simulink model "robot_fis_opt_monte_carlo"  (R2023a)
settings: Solver=FixedStepDiscrete  StartTime=0.0  StopTime=200  RelTol=1e-3
model workspace (MAT data in the model file):
  x = 1
  y = [100; 100; 100; 100; 100; 100; 100; 100; 100; 100; 100; 100; 100; 100; 100; 100; 100; 100; 100; 100; 100; 95; 90; 85; 80; 75; 70; 65; 60; 55; 50; 45; 40; 35; 30; 25; 20; 15; 10; 5; 0; 0; 0; 0; 0; 0; 0; 0; 0; 0; 0; 0; 0; 0; 0; 0; 0; 0; 0; 0; 0; 0; 0; 0; 0; 0; 0; 0; 0; 0; 0; 0; 0; 0; 0; 0; 0; 0; 0; 0; 0; 0; 0; 0; 0; 0; 0; 0; 0; 0; 0; 0; 0; 0; 0; 0; 0; 0; 0; 0; 0; 0; 0; 0; 0; 0; 0; 0; 0; 0; 0; 0; 0; 0; 0; 0; 0; 0; 0; 0; 0; 0; 0; 0; 0; 0; 0; 0; 0; 0; 0; 0; 0; 0; 0; 0; 0; 0; 0; 0; 0; 0; 0; 0; 0; 0; 0; 0; 0; 0; 0; 0; 0; 0; 0; 0; 0; 0; 0; 0; 0; 0; 0; 0; 0; 0; 0; 0; 0; 0; 0; 0; 0; 0; 0; 0; 0; 0; 0; 0; 0; 0; 0; 0; 0; 0; 0; 0; 0; 0; 0; 0; 0; 0; 0; 0; 0; 0; 0; 0; 0; 0; 0; 0; 0; 0; 0; 0; 0; 0; 0; 0; 0; 0; 0; 0; 0; 0; 0; 0; 0; 0; 0; 0; 0; 0; 0; 0; 0; 0; 0; 0; 0; 0; 0; 0; 0; 0; 0; 0; 0; 0; 0; 0; 0; 0; 0; 0; 0; 0; 0; 0; 0; 0; 0; 0]
libraries: fuzblock x1
settings Model: DataTypeOverride=Off  SnapshotBufferSize=1000  SnapshotInterval=1000  Creator=Mohammad  LastModifiedBy=Mohammad
settings SolverCC: AlgebraicLoopSolver=TrustRegion
settings DataIOCC: SaveOutput=off  SaveTime=off
settings OptimizationCC: BlockReduction=off  ConditionallyExecuteInputs=off  DefaultParameterBehavior=Inlined
settings DebuggingCC: AlgebraicLoopMsg=error  SingleTaskRateTransMsg=error  UnconnectedInputMsg=warning  UnconnectedOutputMsg=warning  UnconnectedLineMsg=warning  StrictBusMsg=ErrorOnBusTreatedAsVector  ArithmeticOperatorsInVariantConditions=warning
settings HardwareCC: ProdBitPerPointer=32  ProdBitPerSizeT=32  ProdBitPerPtrDiffT=32  ProdLargestAtomicFloat=None  ProdIntDivRoundTo=Undefined  ProdEndianess=Unspecified  ProdWordSize=32  ProdHWDeviceType=ASIC/FPGA->ASIC/FPGA  ProdEqTarget=off
settings ModelReferenceCC: EnableRefExpFcnMdlSchedulingChecks=on
settings SFSimCC: SimUseLocalCustomCode=off  CustomCodeUndefinedFunction=UseInterfaceOnly
settings RTWCC: RTWUseLocalCustomCode=off
settings CodeAppCC: StateflowObjectComments=on
settings GRTTargetCC: TargetLangStandard=C89/C90 (ANSI)

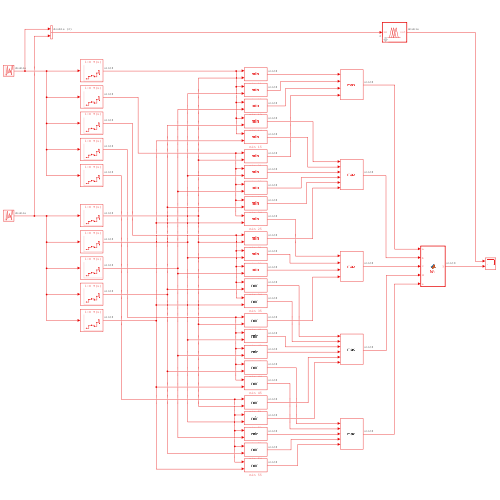
[thumbnail: Simulink's stored preview of the top-level diagram]
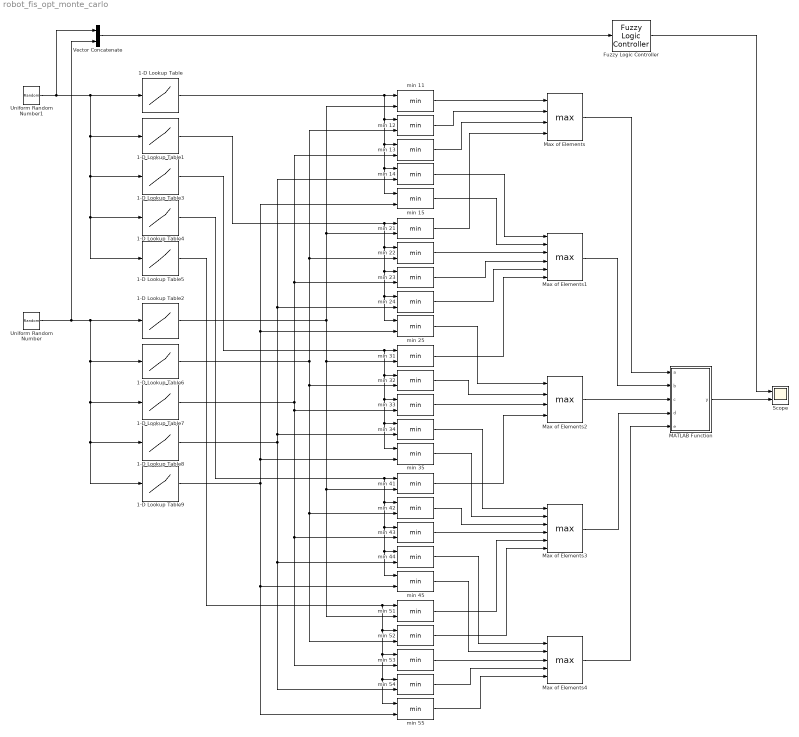
== system robot_fis_opt_monte_carlo ==
  1-D Lookup Table : Lookup_n-D  NumberOfTableDimensions=1  BreakpointsSpecification=Even spacing  BreakpointsForDimension1=[0 1 2 3 4 5 6 7]  BreakpointsForDimension1FirstPoint=0  BreakpointsForDimension1Min=0  BreakpointsForDimension1Max=255  BreakpointsForDimension1DataTypeStr=uint8  IndexSearchMethod=Linear search  Table=[100;100;100;100;100;100;100;100;100;100;100;100;100;100;100;100;100;100;100;100;100;95;90;85;80;75;70;65;64;64;50;45;40;35;30;25;20;15;10;5;0;0;0;0;0;0;0;0;0;0;0;0;0;0;0;0;0;0;0;0;0;0;0;0;0;0;0;0;0;0;0;0;0;0;0;0;0;0;0;0;0;0;0;0;0;0;0;0;0;0;0;0;0;0;0;0;0;0;0;0;0;0;0;0;0;0;0;0;0;0;0;0;0;0;0;0;0;0;0;0;0;0;0;0;0;0;0;0;0;0;0;0;0;0;0;0;0;0;0;0;0;0;0;0;0;0;0;0;0;0;0;0;0;0;0;0;0;0;0;0;0;0;0;0;0;0;0;0;0;0;0;0;0;0;0;0;0;0;0;0;0;0;0;0;0;0;0;0;0;0;0;0;0;0;0;0;0;0;0;0;0;0;0;0;0;0;0;0;0;0;0;0;0;0;0;0;0;0;0;0;0;0;0;0;0;0;0;0;0;0;0;0;0;0;0;0;0;0;0;0;0;0;0;0;0;0;0;0;0;0;0;0;0;0;0;0]  TableMin=0  TableMax=100  TableDataTypeStr=uint8  IntermediateResultsDataTypeStr=int8  InterpMethod=Flat  InternalRulePriority=Speed  OutDataTypeStr=uint8  FractionDataTypeStr=fixdt(0,8,0)
  1-D Lookup Table1 : Lookup_n-D  NumberOfTableDimensions=1  BreakpointsSpecification=Even spacing  BreakpointsForDimension1=[0 1 2 3 4 5 6 7]  BreakpointsForDimension1FirstPoint=0  BreakpointsForDimension1Min=0  BreakpointsForDimension1Max=255  BreakpointsForDimension1DataTypeStr=uint8  IndexSearchMethod=Linear search  Table=[0;0;0;0;0;0;0;0;0;0;0;0;0;0;0;0;0;0;0;0;0;5;10;15;20;25;30;35;40;45;50;55;64;65;70;75;80;85;90;95;100;100;100;100;100;100;100;100;100;100;100;100;100;100;100;100;100;100;100;100;100;95;90;85;80;75;70;65;64;64;50;45;40;35;30;25;20;15;10;5;0;0;0;0;0;0;0;0;0;0;0;0;0;0;0;0;0;0;0;0;0;0;0;0;0;0;0;0;0;0;0;0;0;0;0;0;0;0;0;0;0;0;0;0;0;0;0;0;0;0;0;0;0;0;0;0;0;0;0;0;0;0;0;0;0;0;0;0;0;0;0;0;0;0;0;0;0;0;0;0;0;0;0;0;0;0;0;0;0;0;0;0;0;0;0;0;0;0;0;0;0;0;0;0;0;0;0;0;0;0;0;0;0;0;0;0;0;0;0;0;0;0;0;0;0;0;0;0;0;0;0;0;0;0;0;0;0;0;0;0;0;0;0;0;0;0;0;0;0;0;0;0;0;0;0;0;0;0;0;0;0;0;0;0;0;0;0;0;0;0;0;0;0;0;0;0]  TableMin=0  TableMax=100  TableDataTypeStr=uint8  IntermediateResultsDataTypeStr=int8  InterpMethod=Flat  InternalRulePriority=Speed  OutDataTypeStr=uint8  FractionDataTypeStr=fixdt(0,8,0)
  1-D Lookup Table2 : Lookup_n-D  NumberOfTableDimensions=1  BreakpointsSpecification=Even spacing  BreakpointsForDimension1=[0 1 2 3 4 5 6 7]  BreakpointsForDimension1FirstPoint=0  BreakpointsForDimension1Min=0  BreakpointsForDimension1Max=1023  BreakpointsForDimension1DataTypeStr=fixdt(0,10)  IndexSearchMethod=Linear search  Table=[100;100;100;100;100;100;100;100;100;100;100;100;100;100;100;100;100;100;100;100;100;100;100;100;100;100;100;100;100;100;100;100;100;100;100;100;100;100;100;100;100;100;100;100;100;100;100;100;100;100;100;100;100;100;100;100;100;100;100;100;100;100;100;100;100;100;100;100;100;100;100;100;100;100;100;100;100;100;100;100;100;100;100;100;100;100;100;100;100;100;100;100;100;100;100;100;100;100;100;100;100;99;98;97;96;95;94;93;92;91;90;89;88;87;86;85;84;83;82;81;80;79;78;77;76;75;74;73;63;63;63;63;63;63;63;63;63;63;62;61;60;59;58;57;56;55;54;53;52;51;50;49;48;47;46;45;44;43;42;41;40;39;38;37;36;35;34;33;32;31;30;29;28;27;26;25;24;23;22;21;20;19;18;17;16;15;14;13;12;11;10;9;8;7;6;5;4;3;2;1;0;0;0;0;0;0;0;0;0;0;0;0;0;0;0;0;0;0;0;0;0;0;0;0;0;0;0;0;0;0;0;0;0;0;0;0;0;0;0;0;0;0;0;0;0;0;0;0;0;0;0;0;0;0;0;0;0;0;0;0;0;0;0;0;0;0;0;0;0;0;0;0;0;0;0;0;0;0;0;0;0;0;0;0;0;0;0;0;0;0;0;0;0;0;0;0;0;0;0;0;0;0;0;0;0;0;0;0;0;0;0;0;0;0;0;0;0;0;0;0;0;0;0;0;0;0;0;0;0;0;0;0;0;0;0;0;0;0;0;0;0;0;0;0;0;0;0;0;0;0;0;0;0;0;0;0;0;0;0;0;0;0;0;0;0;0;0;0;0;0;0;0;0;0;0;0;0;0;0;0;0;0;0;0;0;0;0;0;0;0;0;0;0;0;0;0;0;0;0;0;0;0;0;0;0;0;0;0;0;0;0;0;0;0;0;0;0;0;0;0;0;0;0;0;0;0;0;0;0;0;0;0;0;0;0;0;0;0;0;0;0;0;0;0;0;0;0;0;0;0;0;0;0;0;0;0;0;0;0;0;0;0;0;0;0;0;0;0;0;0;0;0;0;0;0;0;0;0;0;0;0;0;0;0;0;0;0;0;0;0;0;0;0;0;0;0;0;0;0;0;0;0;0;0;0;0;0;0;0;0;0;0;0;0;0;0;0;0;0;0;0;0;0;0;0;0;0;0;0;0;0;0;0;0;0;0;0;0;0;0;0;0;0;0;0;0;0;0;0;0;0;0;0;0;0;0;0;0;0;0;0;0;0;0;0;0;0;0;0;0;0;0;0;0;0;0;0;0;0;0;0;0;0;0;0;0;0;0;0;0;0;0;0;0;0;0;0;0;0;0;0;0;0;0;0;0;0;0;0;0;0;0;0;0;0;0;0;0;0;0;0;0;0;0;0;0;0;0;0;0;0;0;0;0;0;0;0;0;0;0;0;0;0;0;0;0;0;0;0;0;0;0;0;0;0;0;0;0;0;0;0;0;0;0;0;0;0;0;0;0;0;0;0;0;0;0;0;0;0;0;0;0;0;0;0;0;0;0;0;0;0;0;0;0;0;0;0;0;0;0;0;0;0;0;0;0;0;0;0;0;0;0;0;0;0;0;0;0;0;0;0;0;0;0;0;0;0;0;0;0;0;0;0;0;0;0;0;0;0;0;0;0;0;0;0;0;0;0;0;0;0;0;0;0;0;0;0;0;0;0;0;0;0;0;0;0;0;0;0;0;0;0;0;0;0;0;0;0;0;0;0;0;0;0;0;0;0;0;0;0;0;0;0;0;0;0;0;0;0;0;0;0;0;0;0;0;0;0;0;0;0;0;0;0;0;0;0;0;0;0;0;0;0;0;0;0;0;0;0;0;0;0;0;0;0;0;0;0;0;0;0;0;0;0;0;0;0;0;0;0;0;0;0;0;0;0;0;0;0;0;0;0;0;0;0;0;0;0;0;0;0;0;0;0;0;0;0;0;0;0;0;0;0;0;0;0;0;0;0;0;0;0;0;0;0;0;0;0;0;0;0;0;0;0;0;0;0;0;0;0;0;0;0;0;0;0;0;0;0;0;0;0;0;0;0;0;0;0;0;0;0;0;0;0;0;0;0;0;0;0;0;0;0;0;0;0;0;0;0;0;0;0;0;0;0;0;0;0;0;0;0;0;0;0;0;0;0;0;0;0;0;0;0;0;0;0;0;0;0;0;0;0;0;0;0;0;0;0;0;0;0;0;0;0;0;0;0;0;0;0;0;0;0;0;0;0;0;0;0;0;0;0;0;0;0;0;0;0;0;0;0;0;0;0]  TableMin=0  TableMax=100  TableDataTypeStr=uint8  IntermediateResultsDataTypeStr=int8  InterpMethod=Flat  InternalRulePriority=Speed  OutDataTypeStr=uint8  FractionDataTypeStr=fixdt(0,8,0)
  1-D Lookup Table3 : Lookup_n-D  NumberOfTableDimensions=1  BreakpointsSpecification=Even spacing  BreakpointsForDimension1=[0 1 2 3 4 5 6 7]  BreakpointsForDimension1FirstPoint=0  BreakpointsForDimension1Min=0  BreakpointsForDimension1Max=255  BreakpointsForDimension1DataTypeStr=uint8  IndexSearchMethod=Linear search  Table=[0;0;0;0;0;0;0;0;0;0;0;0;0;0;0;0;0;0;0;0;0;0;0;0;0;0;0;0;0;0;0;0;0;0;0;0;0;0;0;0;0;0;0;0;0;0;0;0;0;0;0;0;0;0;0;0;0;0;0;0;0;5;10;15;20;25;30;35;40;45;50;55;64;65;70;75;80;85;90;95;100;100;100;100;100;100;100;100;100;100;100;100;100;100;100;100;100;100;100;100;100;95;90;85;80;75;70;65;64;64;50;45;40;35;30;25;20;15;10;5;0;0;0;0;0;0;0;0;0;0;0;0;0;0;0;0;0;0;0;0;0;0;0;0;0;0;0;0;0;0;0;0;0;0;0;0;0;0;0;0;0;0;0;0;0;0;0;0;0;0;0;0;0;0;0;0;0;0;0;0;0;0;0;0;0;0;0;0;0;0;0;0;0;0;0;0;0;0;0;0;0;0;0;0;0;0;0;0;0;0;0;0;0;0;0;0;0;0;0;0;0;0;0;0;0;0;0;0;0;0;0;0;0;0;0;0;0;0;0;0;0;0;0;0;0;0;0;0;0;0;0;0;0;0;0;0]  TableMin=0  TableMax=100  TableDataTypeStr=uint8  IntermediateResultsDataTypeStr=int8  InterpMethod=Flat  InternalRulePriority=Speed  OutDataTypeStr=uint8  FractionDataTypeStr=fixdt(0,8,0)
  1-D Lookup Table4 : Lookup_n-D  NumberOfTableDimensions=1  BreakpointsSpecification=Even spacing  BreakpointsForDimension1=[0 1 2 3 4 5 6 7]  BreakpointsForDimension1FirstPoint=0  BreakpointsForDimension1Min=0  BreakpointsForDimension1Max=255  BreakpointsForDimension1DataTypeStr=uint8  IndexSearchMethod=Linear search  Table=[0;0;0;0;0;0;0;0;0;0;0;0;0;0;0;0;0;0;0;0;0;0;0;0;0;0;0;0;0;0;0;0;0;0;0;0;0;0;0;0;0;0;0;0;0;0;0;0;0;0;0;0;0;0;0;0;0;0;0;0;0;0;0;0;0;0;0;0;0;0;0;0;0;0;0;0;0;0;0;0;0;0;0;0;0;0;0;0;0;0;0;0;0;0;0;0;0;0;0;0;0;5;10;15;20;25;30;35;40;45;50;55;64;65;70;75;80;85;90;95;100;100;100;100;100;100;100;100;100;100;100;100;100;100;100;100;100;100;100;100;100;95;90;85;80;75;70;65;64;64;50;45;40;35;30;25;20;15;10;5;0;0;0;0;0;0;0;0;0;0;0;0;0;0;0;0;0;0;0;0;0;0;0;0;0;0;0;0;0;0;0;0;0;0;0;0;0;0;0;0;0;0;0;0;0;0;0;0;0;0;0;0;0;0;0;0;0;0;0;0;0;0;0;0;0;0;0;0;0;0;0;0;0;0;0;0;0;0;0;0;0;0;0;0;0;0;0;0;0;0;0;0;0;0;0;0]  TableMin=0  TableMax=100  TableDataTypeStr=uint8  IntermediateResultsDataTypeStr=int8  InterpMethod=Flat  InternalRulePriority=Speed  OutDataTypeStr=uint8  FractionDataTypeStr=fixdt(0,8,0)
  1-D Lookup Table5 : Lookup_n-D  NumberOfTableDimensions=1  BreakpointsSpecification=Even spacing  BreakpointsForDimension1=[0 1 2 3 4 5 6 7]  BreakpointsForDimension1FirstPoint=0  BreakpointsForDimension1Min=0  BreakpointsForDimension1Max=255  BreakpointsForDimension1DataTypeStr=uint8  IndexSearchMethod=Linear search  Table=[0;0;0;0;0;0;0;0;0;0;0;0;0;0;0;0;0;0;0;0;0;0;0;0;0;0;0;0;0;0;0;0;0;0;0;0;0;0;0;0;0;0;0;0;0;0;0;0;0;0;0;0;0;0;0;0;0;0;0;0;0;0;0;0;0;0;0;0;0;0;0;0;0;0;0;0;0;0;0;0;0;0;0;0;0;0;0;0;0;0;0;0;0;0;0;0;0;0;0;0;0;0;0;0;0;0;0;0;0;0;0;0;0;0;0;0;0;0;0;0;0;0;0;0;0;0;0;0;0;0;0;0;0;0;0;0;0;0;0;0;0;5;10;15;32;32;32;35;40;45;50;55;60;65;70;75;80;85;90;95;100;100;100;100;100;100;100;100;100;100;100;100;100;100;100;100;100;100;100;100;100;100;100;100;100;100;100;100;100;100;100;100;100;100;100;100;100;100;100;100;100;100;100;100;100;100;100;100;100;100;100;100;100;100;100;100;100;100;100;100;100;100;100;100;100;100;100;100;100;100;100;100;100;100;100;100;100;100;100;100;100;100;100;100;100;100;100;100;100;100;100;100;100;100;100;100]  TableMin=0  TableMax=100  TableDataTypeStr=uint8  IntermediateResultsDataTypeStr=int8  InterpMethod=Flat  InternalRulePriority=Speed  OutDataTypeStr=uint8  FractionDataTypeStr=fixdt(0,8,0)
  1-D Lookup Table6 : Lookup_n-D  NumberOfTableDimensions=1  BreakpointsSpecification=Even spacing  BreakpointsForDimension1=[0 1 2 3 4 5 6 7]  BreakpointsForDimension1FirstPoint=0  BreakpointsForDimension1Min=0  BreakpointsForDimension1Max=1023  BreakpointsForDimension1DataTypeStr=fixdt(0,10)  IndexSearchMethod=Linear search  Table=[0;0;0;0;0;0;0;0;0;0;0;0;0;0;0;0;0;0;0;0;0;0;0;0;0;0;0;0;0;0;0;0;0;0;0;0;0;0;0;0;0;0;0;0;0;0;0;0;0;0;0;0;0;0;0;0;0;0;0;0;0;0;0;0;0;0;0;0;0;0;0;0;0;0;0;0;0;0;0;0;0;0;0;0;0;0;0;0;0;0;0;0;0;0;0;0;0;0;0;0;0;1;2;3;4;5;6;7;8;9;10;11;12;13;14;15;16;17;18;19;20;21;22;23;24;25;26;27;28;29;30;31;32;33;34;35;36;37;38;39;40;41;42;43;44;45;46;47;48;49;50;51;52;53;54;55;56;57;58;59;64;64;64;64;64;65;66;67;68;69;70;71;72;73;74;75;76;77;78;79;80;81;82;83;84;85;86;87;88;89;90;91;92;93;94;95;96;97;98;99;100;100;100;100;100;100;100;100;100;100;100;100;100;100;100;100;100;100;100;100;100;100;100;100;100;100;100;100;100;100;100;100;100;100;100;100;100;100;100;100;100;100;100;100;100;100;100;100;100;100;100;100;100;100;100;100;100;100;100;100;100;100;100;100;100;100;100;100;100;100;100;100;100;100;100;100;100;100;100;100;100;100;100;100;100;100;100;100;100;100;100;100;100;100;100;100;100;100;100;100;100;99;98;97;96;95;94;93;92;91;90;89;88;87;86;85;84;83;82;81;80;79;78;77;76;75;74;73;72;71;70;69;68;67;66;65;64;64;64;64;64;64;64;64;64;64;64;64;64;64;64;64;48;47;46;45;44;43;42;41;40;39;38;37;36;35;34;33;32;31;30;29;28;27;26;25;24;23;22;21;20;19;18;17;16;15;14;13;12;11;10;9;8;7;6;5;4;3;2;1;0;0;0;0;0;0;0;0;0;0;0;0;0;0;0;0;0;0;0;0;0;0;0;0;0;0;0;0;0;0;0;0;0;0;0;0;0;0;0;0;0;0;0;0;0;0;0;0;0;0;0;0;0;0;0;0;0;0;0;0;0;0;0;0;0;0;0;0;0;0;0;0;0;0;0;0;0;0;0;0;0;0;0;0;0;0;0;0;0;0;0;0;0;0;0;0;0;0;0;0;0;0;0;0;0;0;0;0;0;0;0;0;0;0;0;0;0;0;0;0;0;0;0;0;0;0;0;0;0;0;0;0;0;0;0;0;0;0;0;0;0;0;0;0;0;0;0;0;0;0;0;0;0;0;0;0;0;0;0;0;0;0;0;0;0;0;0;0;0;0;0;0;0;0;0;0;0;0;0;0;0;0;0;0;0;0;0;0;0;0;0;0;0;0;0;0;0;0;0;0;0;0;0;0;0;0;0;0;0;0;0;0;0;0;0;0;0;0;0;0;0;0;0;0;0;0;0;0;0;0;0;0;0;0;0;0;0;0;0;0;0;0;0;0;0;0;0;0;0;0;0;0;0;0;0;0;0;0;0;0;0;0;0;0;0;0;0;0;0;0;0;0;0;0;0;0;0;0;0;0;0;0;0;0;0;0;0;0;0;0;0;0;0;0;0;0;0;0;0;0;0;0;0;0;0;0;0;0;0;0;0;0;0;0;0;0;0;0;0;0;0;0;0;0;0;0;0;0;0;0;0;0;0;0;0;0;0;0;0;0;0;0;0;0;0;0;0;0;0;0;0;0;0;0;0;0;0;0;0;0;0;0;0;0;0;0;0;0;0;0;0;0;0;0;0;0;0;0;0;0;0;0;0;0;0;0;0;0;0;0;0;0;0;0;0;0;0;0;0;0;0;0;0;0;0;0;0;0;0;0;0;0;0;0;0;0;0;0;0;0;0;0;0;0;0;0;0;0;0;0;0;0;0;0;0;0;0;0;0;0;0;0;0;0;0;0;0;0;0;0;0;0;0;0;0;0;0;0;0;0;0;0;0;0;0;0;0;0;0;0;0;0;0;0;0;0;0;0;0;0;0;0;0;0;0;0;0;0;0;0;0;0;0;0;0;0;0;0;0;0;0;0;0;0;0;0;0;0;0;0;0;0;0;0;0;0;0;0;0;0;0;0;0;0;0;0;0;0;0;0;0;0;0;0;0;0;0;0;0;0;0;0;0;0;0;0;0;0;0;0;0;0;0;0;0;0;0;0;0;0;0;0;0;0;0;0;0;0;0;0;0;0;0;0;0;0;0;0;0;0;0;0;0;0;0;0;0;0;0;0;0;0;0;0;0;0;0;0;0;0;0;0;0;0;0;0;0;0;0;0;0;0;0;0;0;0;0;0;0;0;0;0;0;0]  TableMin=0  TableMax=100  TableDataTypeStr=uint8  IntermediateResultsDataTypeStr=int8  InterpMethod=Flat  InternalRulePriority=Speed  OutDataTypeStr=uint8  FractionDataTypeStr=fixdt(0,8,0)
  1-D Lookup Table7 : Lookup_n-D  NumberOfTableDimensions=1  BreakpointsSpecification=Even spacing  BreakpointsForDimension1=[0 1 2 3 4 5 6 7]  BreakpointsForDimension1FirstPoint=0  BreakpointsForDimension1Min=0  BreakpointsForDimension1Max=1023  BreakpointsForDimension1DataTypeStr=fixdt(0,10)  IndexSearchMethod=Linear search  Table=[0;0;0;0;0;0;0;0;0;0;0;0;0;0;0;0;0;0;0;0;0;0;0;0;0;0;0;0;0;0;0;0;0;0;0;0;0;0;0;0;0;0;0;0;0;0;0;0;0;0;0;0;0;0;0;0;0;0;0;0;0;0;0;0;0;0;0;0;0;0;0;0;0;0;0;0;0;0;0;0;0;0;0;0;0;0;0;0;0;0;0;0;0;0;0;0;0;0;0;0;0;0;0;0;0;0;0;0;0;0;0;0;0;0;0;0;0;0;0;0;0;0;0;0;0;0;0;0;0;0;0;0;0;0;0;0;0;0;0;0;0;0;0;0;0;0;0;0;0;0;0;0;0;0;0;0;0;0;0;0;0;0;0;0;0;0;0;0;0;0;0;0;0;0;0;0;0;0;0;0;0;0;0;0;0;0;0;0;0;0;0;0;0;0;0;0;0;0;0;0;0;0;0;0;0;0;0;0;0;0;0;0;0;0;0;0;0;0;0;0;0;0;0;0;0;0;0;0;0;0;0;0;0;0;0;0;0;0;0;0;0;0;0;0;0;0;0;0;0;0;0;0;0;0;0;0;0;0;0;0;0;0;0;0;0;0;0;0;0;0;0;0;0;0;0;0;0;0;0;0;0;0;0;0;0;0;0;0;0;0;0;0;0;0;0;0;0;0;0;0;0;1;2;3;4;5;6;7;8;9;10;11;12;13;14;15;16;17;18;19;20;21;22;23;24;25;26;27;28;29;30;31;32;33;34;35;36;37;38;39;40;41;42;43;44;45;46;47;48;49;50;51;64;64;64;64;64;64;64;64;64;64;64;64;64;65;66;67;68;69;70;71;72;73;74;75;76;77;78;79;80;81;82;83;84;85;86;87;88;89;90;91;92;93;94;95;96;97;98;99;100;100;100;100;100;100;100;100;100;100;100;100;100;100;100;100;100;100;100;100;100;100;100;100;100;100;100;100;100;100;100;100;100;100;100;100;100;100;100;100;100;100;100;100;100;100;100;100;100;100;100;100;100;100;100;100;100;100;100;100;100;100;100;100;100;100;100;100;100;100;100;100;100;100;100;100;100;100;100;100;100;100;100;100;100;100;100;100;100;100;100;100;100;100;100;100;100;100;100;100;100;99;98;97;96;95;94;93;92;91;90;89;88;87;86;85;84;83;82;81;80;79;78;77;76;75;74;73;72;71;70;69;68;67;66;65;64;64;64;64;64;64;64;64;56;55;54;53;52;51;50;49;48;47;46;45;44;43;42;41;40;39;38;37;36;35;34;33;32;31;30;29;28;27;26;25;24;23;22;21;20;19;18;17;16;15;14;13;12;11;10;9;8;7;6;5;4;3;2;1;0;0;0;0;0;0;0;0;0;0;0;0;0;0;0;0;0;0;0;0;0;0;0;0;0;0;0;0;0;0;0;0;0;0;0;0;0;0;0;0;0;0;0;0;0;0;0;0;0;0;0;0;0;0;0;0;0;0;0;0;0;0;0;0;0;0;0;0;0;0;0;0;0;0;0;0;0;0;0;0;0;0;0;0;0;0;0;0;0;0;0;0;0;0;0;0;0;0;0;0;0;0;0;0;0;0;0;0;0;0;0;0;0;0;0;0;0;0;0;0;0;0;0;0;0;0;0;0;0;0;0;0;0;0;0;0;0;0;0;0;0;0;0;0;0;0;0;0;0;0;0;0;0;0;0;0;0;0;0;0;0;0;0;0;0;0;0;0;0;0;0;0;0;0;0;0;0;0;0;0;0;0;0;0;0;0;0;0;0;0;0;0;0;0;0;0;0;0;0;0;0;0;0;0;0;0;0;0;0;0;0;0;0;0;0;0;0;0;0;0;0;0;0;0;0;0;0;0;0;0;0;0;0;0;0;0;0;0;0;0;0;0;0;0;0;0;0;0;0;0;0;0;0;0;0;0;0;0;0;0;0;0;0;0;0;0;0;0;0;0;0;0;0;0;0;0;0;0;0;0;0;0;0;0;0;0;0;0;0;0;0;0;0;0;0;0;0;0;0;0;0;0;0;0;0;0;0;0;0;0;0;0;0;0;0;0;0;0;0;0;0;0;0;0;0;0;0;0;0;0;0;0;0;0;0;0;0;0;0;0;0;0;0;0;0;0;0;0;0;0;0;0;0;0;0;0;0;0;0;0;0;0;0;0;0;0;0;0;0;0;0;0;0;0;0;0;0;0;0;0;0;0;0;0;0;0;0;0;0;0;0;0;0;0;0;0;0;0;0;0;0;0;0;0;0;0;0;0;0;0;0;0;0;0;0;0;0;0;0;0;0;0;0;0]  TableMin=0  TableMax=100  TableDataTypeStr=uint8  IntermediateResultsDataTypeStr=int8  InterpMethod=Flat  InternalRulePriority=Speed  OutDataTypeStr=uint8  FractionDataTypeStr=fixdt(0,8,0)
  1-D Lookup Table8 : Lookup_n-D  NumberOfTableDimensions=1  BreakpointsSpecification=Even spacing  BreakpointsForDimension1=[0 1 2 3 4 5 6 7]  BreakpointsForDimension1FirstPoint=0  BreakpointsForDimension1Min=0  BreakpointsForDimension1Max=1023  BreakpointsForDimension1DataTypeStr=fixdt(0,10)  IndexSearchMethod=Linear search  Table=[0;0;0;0;0;0;0;0;0;0;0;0;0;0;0;0;0;0;0;0;0;0;0;0;0;0;0;0;0;0;0;0;0;0;0;0;0;0;0;0;0;0;0;0;0;0;0;0;0;0;0;0;0;0;0;0;0;0;0;0;0;0;0;0;0;0;0;0;0;0;0;0;0;0;0;0;0;0;0;0;0;0;0;0;0;0;0;0;0;0;0;0;0;0;0;0;0;0;0;0;0;0;0;0;0;0;0;0;0;0;0;0;0;0;0;0;0;0;0;0;0;0;0;0;0;0;0;0;0;0;0;0;0;0;0;0;0;0;0;0;0;0;0;0;0;0;0;0;0;0;0;0;0;0;0;0;0;0;0;0;0;0;0;0;0;0;0;0;0;0;0;0;0;0;0;0;0;0;0;0;0;0;0;0;0;0;0;0;0;0;0;0;0;0;0;0;0;0;0;0;0;0;0;0;0;0;0;0;0;0;0;0;0;0;0;0;0;0;0;0;0;0;0;0;0;0;0;0;0;0;0;0;0;0;0;0;0;0;0;0;0;0;0;0;0;0;0;0;0;0;0;0;0;0;0;0;0;0;0;0;0;0;0;0;0;0;0;0;0;0;0;0;0;0;0;0;0;0;0;0;0;0;0;0;0;0;0;0;0;0;0;0;0;0;0;0;0;0;0;0;0;0;0;0;0;0;0;0;0;0;0;0;0;0;0;0;0;0;0;0;0;0;0;0;0;0;0;0;0;0;0;0;0;0;0;0;0;0;0;0;0;0;0;0;0;0;0;0;0;0;0;0;0;0;0;0;0;0;0;0;0;0;0;0;0;0;0;0;0;0;0;0;0;0;0;0;0;0;0;0;0;0;0;0;0;0;0;0;0;0;0;0;0;0;0;0;0;0;0;0;0;0;0;0;0;0;0;0;0;0;0;0;0;0;0;0;0;0;0;0;0;0;0;0;0;0;0;0;0;0;0;0;0;0;0;0;0;0;0;0;0;0;0;0;0;0;0;0;0;0;0;0;0;0;0;0;0;0;0;0;0;0;0;0;0;0;0;0;0;0;0;0;0;0;0;0;0;0;0;0;0;0;0;0;0;0;0;0;0;0;0;0;0;0;0;0;0;0;0;0;0;1;2;3;4;5;6;7;8;9;10;11;12;13;14;15;16;17;18;19;20;21;22;23;24;25;26;27;28;29;30;31;32;33;34;35;36;37;38;39;40;41;42;43;44;45;46;47;48;49;50;51;52;53;54;55;56;57;58;59;60;61;62;63;63;63;63;63;63;63;63;63;63;63;63;63;76;77;78;79;80;81;82;83;84;85;86;87;88;89;90;91;92;93;94;95;96;97;98;99;100;100;100;100;100;100;100;100;100;100;100;100;100;100;100;100;100;100;100;100;100;100;100;100;100;100;100;100;100;100;100;100;100;100;100;100;100;100;100;100;100;100;100;100;100;100;100;100;100;100;100;100;100;100;100;100;100;100;100;100;100;100;100;100;100;100;100;100;100;100;100;100;100;100;100;100;100;100;100;100;100;100;100;100;100;100;100;100;100;100;100;100;100;100;100;100;100;100;100;100;100;99;98;97;96;95;94;93;92;91;90;89;88;87;86;85;84;83;82;81;80;79;78;77;76;75;74;73;72;71;70;69;68;67;66;65;63;63;62;61;60;59;58;57;56;55;54;53;52;51;50;49;48;47;46;45;44;43;42;41;40;39;38;37;36;35;34;33;32;31;30;29;28;27;26;25;24;23;22;21;20;19;18;17;16;15;14;13;12;11;10;9;8;7;6;5;4;3;2;1;0;0;0;0;0;0;0;0;0;0;0;0;0;0;0;0;0;0;0;0;0;0;0;0;0;0;0;0;0;0;0;0;0;0;0;0;0;0;0;0;0;0;0;0;0;0;0;0;0;0;0;0;0;0;0;0;0;0;0;0;0;0;0;0;0;0;0;0;0;0;0;0;0;0;0;0;0;0;0;0;0;0;0;0;0;0;0;0;0;0;0;0;0;0;0;0;0;0;0;0;0;0;0;0;0;0;0;0;0;0;0;0;0;0;0;0;0;0;0;0;0;0;0;0;0;0;0;0;0;0;0;0;0;0;0;0;0;0;0;0;0;0;0;0;0;0;0;0;0;0;0;0;0;0;0;0;0;0;0;0;0;0;0;0;0;0;0;0;0;0;0;0;0;0;0;0;0;0;0;0;0;0;0;0;0;0;0;0;0;0;0;0;0;0;0;0;0;0;0;0;0;0;0;0;0;0;0;0;0;0;0;0;0;0;0;0;0;0;0;0;0;0;0;0]  TableMin=0  TableMax=100  TableDataTypeStr=uint8  IntermediateResultsDataTypeStr=int8  InterpMethod=Flat  InternalRulePriority=Speed  OutDataTypeStr=uint8  FractionDataTypeStr=fixdt(0,8,0)
  1-D Lookup Table9 : Lookup_n-D  NumberOfTableDimensions=1  BreakpointsSpecification=Even spacing  BreakpointsForDimension1=[0 1 2 3 4 5 6 7]  BreakpointsForDimension1FirstPoint=0  BreakpointsForDimension1Min=0  BreakpointsForDimension1Max=1023  BreakpointsForDimension1DataTypeStr=fixdt(0,10)  IndexSearchMethod=Linear search  Table=[0;0;0;0;0;0;0;0;0;0;0;0;0;0;0;0;0;0;0;0;0;0;0;0;0;0;0;0;0;0;0;0;0;0;0;0;0;0;0;0;0;0;0;0;0;0;0;0;0;0;0;0;0;0;0;0;0;0;0;0;0;0;0;0;0;0;0;0;0;0;0;0;0;0;0;0;0;0;0;0;0;0;0;0;0;0;0;0;0;0;0;0;0;0;0;0;0;0;0;0;0;0;0;0;0;0;0;0;0;0;0;0;0;0;0;0;0;0;0;0;0;0;0;0;0;0;0;0;0;0;0;0;0;0;0;0;0;0;0;0;0;0;0;0;0;0;0;0;0;0;0;0;0;0;0;0;0;0;0;0;0;0;0;0;0;0;0;0;0;0;0;0;0;0;0;0;0;0;0;0;0;0;0;0;0;0;0;0;0;0;0;0;0;0;0;0;0;0;0;0;0;0;0;0;0;0;0;0;0;0;0;0;0;0;0;0;0;0;0;0;0;0;0;0;0;0;0;0;0;0;0;0;0;0;0;0;0;0;0;0;0;0;0;0;0;0;0;0;0;0;0;0;0;0;0;0;0;0;0;0;0;0;0;0;0;0;0;0;0;0;0;0;0;0;0;0;0;0;0;0;0;0;0;0;0;0;0;0;0;0;0;0;0;0;0;0;0;0;0;0;0;0;0;0;0;0;0;0;0;0;0;0;0;0;0;0;0;0;0;0;0;0;0;0;0;0;0;0;0;0;0;0;0;0;0;0;0;0;0;0;0;0;0;0;0;0;0;0;0;0;0;0;0;0;0;0;0;0;0;0;0;0;0;0;0;0;0;0;0;0;0;0;0;0;0;0;0;0;0;0;0;0;0;0;0;0;0;0;0;0;0;0;0;0;0;0;0;0;0;0;0;0;0;0;0;0;0;0;0;0;0;0;0;0;0;0;0;0;0;0;0;0;0;0;0;0;0;0;0;0;0;0;0;0;0;0;0;0;0;0;0;0;0;0;0;0;0;0;0;0;0;0;0;0;0;0;0;0;0;0;0;0;0;0;0;0;0;0;0;0;0;0;0;0;0;0;0;0;0;0;0;0;0;0;0;0;0;0;0;0;0;0;0;0;0;0;0;0;0;0;0;0;0;0;0;0;0;0;0;0;0;0;0;0;0;0;0;0;0;0;0;0;0;0;0;0;0;0;0;0;0;0;0;0;0;0;0;0;0;0;0;0;0;0;0;0;0;0;0;0;0;0;0;0;0;0;0;0;0;0;0;0;0;0;0;0;0;0;0;0;0;0;0;0;0;0;0;0;0;0;0;0;0;0;0;0;0;0;0;0;0;0;0;0;0;0;0;0;0;0;0;0;0;0;0;0;0;0;0;0;0;0;0;0;0;0;0;0;0;0;0;0;0;0;0;0;0;0;0;0;0;0;0;0;0;0;0;0;0;0;0;0;0;0;0;0;0;0;0;0;0;0;0;0;0;0;0;0;0;0;0;0;0;0;0;0;0;0;0;0;0;0;0;0;0;0;0;0;0;0;0;0;0;0;0;0;0;0;0;0;0;0;0;0;0;0;0;0;0;0;0;1;2;3;4;5;6;7;8;9;10;11;12;13;14;15;16;17;18;19;20;21;22;23;24;25;26;27;28;29;30;31;32;33;34;35;36;37;38;39;40;41;42;43;44;45;46;47;48;49;50;51;52;53;54;55;56;57;58;59;60;61;62;63;63;63;63;63;68;69;70;71;72;73;74;75;76;77;78;79;80;81;82;83;84;85;86;87;88;89;90;91;92;93;94;95;96;97;98;99;100;100;100;100;100;100;100;100;100;100;100;100;100;100;100;100;100;100;100;100;100;100;100;100;100;100;100;100;100;100;100;100;100;100;100;100;100;100;100;100;100;100;100;100;100;100;100;100;100;100;100;100;100;100;100;100;100;100;100;100;100;100;100;100;100;100;100;100;100;100;100;100;100;100;100;100;100;100;100;100;100;100;100;100;100;100;100;100;100;100;100;100;100;100;100;100;100;100;100;100;100;100;100;100;100;100;100;100;100;100;100;100;100;100;100;100;100;100;100;100;100;100;100;100;100;100;100;100;100;100;100;100;100;100;100;100;100;100;100;100;100;100;100;100;100;100;100;100;100;100;100;100;100;100;100;100;100;100;100;100;100;100;100;100;100;100;100;100;100;100;100;100;100;100;100;100;100;100;100;100;100;100;100;100;100;100;100;100;100;100;100;100;100;100;100;100;100;100;100;100;100;100;100;100;100;100;100;100;100;100;100;100;100;100;100;100;100;100;100;100;100;100;100;100]  TableMin=0  TableMax=100  TableDataTypeStr=uint8  IntermediateResultsDataTypeStr=int8  InterpMethod=Flat  InternalRulePriority=Speed  OutDataTypeStr=uint8  FractionDataTypeStr=fixdt(0,8,0)
  Fuzzy Logic Controller : fuzblock/Fuzzy Logic  Controller  FIS=robot  OutputSampleNumber=101  DataType=double  FuzzifiedInputs=off  RuleFiringStrengths=off  RuleOutputs=off  AggregatedOutputs=off  SimulateUsing=Interpreted execution  OutOfRangeInputValueMessage=warning  NoRuleFiredMessage=warning  EmptyOutputFuzzySetMessage=warning
  MATLAB Function : MATLAB Function  TreatAsAtomicUnit=on
  Max of Elements : MinMax  Function=max  Inputs=4  OutMin=0  OutMax=100  OutDataTypeStr=uint8
  Max of Elements1 : MinMax  Function=max  Inputs=6  OutDataTypeStr=uint8
  Max of Elements2 : MinMax  Function=max  Inputs=4  OutDataTypeStr=uint8
  Max of Elements3 : MinMax  Function=max  Inputs=6  OutDataTypeStr=uint8
  Max of Elements4 : MinMax  Function=max  Inputs=5  OutDataTypeStr=uint8
  Scope : Scope  NumInputPorts=2
  Uniform Random Number : UniformRandomNumber  Minimum=0  Maximum=1023  Seed=49  SampleTime=1
  Uniform Random Number1 : UniformRandomNumber  Minimum=0  Maximum=180  Seed=23  SampleTime=1
  Vector Concatenate : Concatenate
  min {11..15,21..25,31..35,41..45,51..55} (25 alike) : MinMax  Inputs=2  OutMin=0  OutMax=100  OutDataTypeStr=uint8
  wires:
  Uniform Random Number/1 -> Vector Concatenate/2, 1-D Lookup Table9/1, 1-D Lookup Table8/1, 1-D Lookup Table7/1, 1-D Lookup Table6/1, 1-D Lookup Table2/1
  Uniform Random Number1/1 -> Vector Concatenate/1, 1-D Lookup Table5/1, 1-D Lookup Table4/1, 1-D Lookup Table3/1, 1-D Lookup Table1/1, 1-D Lookup Table/1
  1-D Lookup Table/1 -> min 11/1, min 12/1, min 13/1, min 15/1, min 14/1
  1-D Lookup Table2/1 -> min 31/2, min 51/2, min 41/2, min 21/2, min 11/2
  1-D Lookup Table1/1 -> min 21/1, min 22/1, min 23/1, min 25/1, min 24/1
  1-D Lookup Table5/1 -> min 51/1, min 52/1, min 53/1, min 55/1, min 54/1
  1-D Lookup Table4/1 -> min 41/1, min 42/1, min 43/1, min 45/1, min 44/1
  1-D Lookup Table3/1 -> min 31/1, min 32/1, min 33/1, min 35/1, min 34/1
  1-D Lookup Table6/1 -> min 32/2, min 52/2, min 42/2, min 22/2, min 12/2
  1-D Lookup Table7/1 -> min 33/2, min 53/2, min 43/2, min 23/2, min 13/2
  1-D Lookup Table8/1 -> min 54/2, min 44/2, min 34/2, min 24/2, min 14/2
  1-D Lookup Table9/1 -> min 55/2, min 45/2, min 35/2, min 25/2, min 15/2
  min 11/1 -> Max of Elements/1
  min 12/1 -> Max of Elements/2
  min 13/1 -> Max of Elements/3
  min 21/1 -> Max of Elements/4
  min 14/1 -> Max of Elements1/1
  min 15/1 -> Max of Elements1/2
  min 22/1 -> Max of Elements1/3
  min 23/1 -> Max of Elements1/4
  min 24/1 -> Max of Elements1/5
  min 31/1 -> Max of Elements1/6
  min 25/1 -> Max of Elements2/1
  min 32/1 -> Max of Elements2/2
  min 33/1 -> Max of Elements2/3
  min 41/1 -> Max of Elements2/4
  min 34/1 -> Max of Elements3/1
  min 35/1 -> Max of Elements3/2
  min 44/1 -> Max of Elements4/1
  min 45/1 -> Max of Elements4/2
  min 53/1 -> Max of Elements4/3
  min 54/1 -> Max of Elements4/4
  min 42/1 -> Max of Elements3/3
  min 43/1 -> Max of Elements3/4
  min 51/1 -> Max of Elements3/5
  min 52/1 -> Max of Elements3/6
  min 55/1 -> Max of Elements4/5
  Max of Elements/1 -> MATLAB Function/1(a)
  Max of Elements1/1 -> MATLAB Function/2(b)
  Max of Elements2/1 -> MATLAB Function/3(c)
  Max of Elements3/1 -> MATLAB Function/4(d)
  Max of Elements4/1 -> MATLAB Function/5(e)
  MATLAB Function/1(y) -> Scope/2
  Vector Concatenate/1 -> Fuzzy Logic Controller/1
  Fuzzy Logic Controller/1 -> Scope/1

== matlab function robot_fis_opt_monte_carlo/MATLAB Function ==
  data: a input; y output; b input; c input; d input; e input
function y = fcn(a,b,c,d,e)
max = a;
y = uint8(0);
if (b >= max)
    max = b;
    y = uint8(1);
end
if (c >= max)
    max = c;
    y = uint8(2);
end
if (d >= max)
    max = d;
    y = uint8(3);
end
if (e >= max)
    y = uint8(4);
end
